simulink model "CM690A_HwAg0Meas"  (R2013b)
settings: Solver=FixedStepDiscrete  SolverMode=SingleTasking  StartTime=0.0  StopTime=22  FixedStep=0.002  RelTol=1e-3
undefined symbols (not defined in the file): ELECGLBPRM_DEGPERREV_DEGPERREV_F32, ELECGLBPRM_HWAGCENTROFFS_HWDEG_F32, ELECGLBPRM_HWAGSATNLOWRLIM_HWDEG_F32, ELECGLBPRM_HWAGSATNUPPRLIM_HWDEG_F32, ELECGLBPRM_HWAGSCA_ULS_F32, ELECGLBPRM_HWAGSPURGEARRAT_ULS_F32, ELECGLBPRM_HWAGSPURTORINGGEARRATSNSR0_ULS_F32, ELECGLBPRM_HWAGSPURTORINGGEARRATSNSR1_ULS_F32, ELECGLBPRM_NOFLT_CNT_U08, ELECGLBPRM_OFFSTRIMNOTPRFMD_CNT_U08, ELECGLBPRM_PRTCLFLT_CNT_U08, ELECGLBPRM_SKIPSTEPFLT_CNT_U08, ELECGLBPRM_SNSRINTFLT_CNT_U08, ELECGLBPRM_VRNRERRFLT_CNT_U08, FLTINJ_HWAG0MEAS_HWAG0, FLTINJ_HWAG0MEAS_TESTOK, HwAg0IfFlt, HwAg0MeasHwAg0IfFltFailStep, HwAg0MeasHwAg0IfFltPassStep, HwAg0MeasHwAg0Snsr0PrtclFltFailStep, HwAg0MeasHwAg0Snsr0PrtclFltPassStep, HwAg0MeasHwAg0Snsr1PrtclFltFailStep, HwAg0MeasHwAg0Snsr1PrtclFltPassStep, HwAg0MeasSnsr0Rev, HwAg0MeasSnsr1Rev, HwAg0MeasStep, HwAg0MeasVrnrErrThd, HwAg0MfgFlt, HwAg0Snsr0PrtclFlt, HwAg0Snsr1PrtclFlt, HWAG10THTOOTHTRIG_CNT_U08, HWAG11THTOOTHTRIG_CNT_U08, NtcSts1, sigbuilder_block, SigQlfr1
libraries: simulink x30, NxtrNvM x3
(part 1 of 5)
settings Model: Creator=CZ68DS  LastModifiedBy=CZ68DS
settings SolverCC: PositivePriorityOrder=on  AutoInsertRateTranBlk=on  InsertRTBMode=Always
settings DataIOCC: LimitDataPoints=off  SaveFormat=Structure  ReturnWorkspaceOutputs=on
settings OptimizationCC: BlockReduction=off  InlineParams=on  ZeroExternalMemoryAtStartup=off  ZeroInternalMemoryAtStartup=off  OptimizeModelRefInitCode=on  LifeSpan=1
settings DebuggingCC: SignalInfNanChecking=error  SignalRangeChecking=warning  ReadBeforeWriteMsg=EnableAllAsWarning  WriteAfterWriteMsg=EnableAllAsWarning  WriteAfterReadMsg=EnableAllAsWarning  UnderspecifiedInitializationDetection=Simplified  MergeDetectMultiDrivingBlocksExec=error  SolverPrmCheckMsg=error  InheritedTsInSrcMsg=error  MultiTaskDSMMsg=warning  SingleTaskRateTransMsg=error  TasksWithSamePriorityMsg=error  SigSpecEnsureSampleTimeMsg=error  CheckMatrixSingularityMsg=error  ParameterUnderflowMsg=error  ParameterPrecisionLossMsg=error  ParameterTunabilityLossMsg=error  FixptConstUnderflowMsg=warning  FixptConstOverflowMsg=warning  FixptConstPrecisionLossMsg=warning  VectorMatrixConversionMsg=error  SignalLabelMismatchMsg=error  UnconnectedInputMsg=error  UnconnectedOutputMsg=error  UnconnectedLineMsg=error  SFcnCompatibilityMsg=error  FrameProcessingCompatibilityMsg=error  UniqueDataStoreMsg=warning  BusObjectLabelMismatch=error  RootOutportRequireBusObject=error  AssertControl=DisableAll  ModelReferenceIOMsg=error  ModelReferenceVersionMismatchMessage=warning  ModelReferenceIOMismatchMessage=error  ModelReferenceDataLoggingMessage=error  StateNameClashWarn=warning  StrictBusMsg=ErrorOnBusTreatedAsVector  NonBusSignalsTreatedAsBus=error  SFUnexpectedBacktrackingDiag=error  SFInvalidInputDataAccessInChartInitDiag=error  SFNoUnconditionalDefaultTransitionDiag=error  SFTransitionOutsideNaturalParentDiag=error  SFUnconditionalTransitionShadowingDiag=error  SFUndirectedBroadcastEventsDiag=error
settings HardwareCC: ProdEndianess=LittleEndian  ProdHWDeviceType=Texas Instruments->TMS470
settings ModelReferenceCC: ModelReferenceNumInstancesAllowed=Single
settings RTWCC: SystemTargetFile=autosar.tlc  GenCodeOnly=on  TemplateMakefile=ert_default_tmf  Description=AUTOSAR  GenerateReport=on  ProcessScript=autosar_make_rtw_hook  LaunchReport=on
settings CodeAppCC: GenerateComments=off  IgnoreCustomStorageClasses=off  CustomSymbolStrType=$N$R$M  CustomSymbolStrBlkIO=$N$M  SimulinkBlockComments=off
settings STFCustomTargetCC: CodeReplacementLibrary=C89/C90 (ANSI)  ParMdlRefBuildCompliant=on  CompOptLevelCompliant=on  IncludeMdlTerminateFcn=off  CombineOutputUpdateFcns=on  SuppressErrorStatus=on  ERTFirstTimeCompliant=on  ERTCustomFileBanners=on  SupportNonFinite=off  SupportComplex=off  SupportContinuousTime=off  SupportNonInlinedSFcns=off  MATLABClassNameForMDSCustomization=Simulink.SoftwareTarget.ERTCustomization  AutosarCompliant=on  GRTInterface=off  SystemTargetFile=autosar.tlc
settings ERTTargetCC: CodeReplacementLibrary=C89/C90 (ANSI)  ConcurrentExecutionCompliant=off  IncludeMdlTerminateFcn=off  SuppressErrorStatus=on  SupportNonFinite=off  SupportComplex=off  ModelStepFunctionPrototypeControlCompliant=off  CPPClassGenCompliant=off  AutosarCompliant=on  InlinedParameterPlacement=NonHierarchical  ERTCustomFileTemplate=example_file_process.tlc  EnableUserReplacementTypes=on

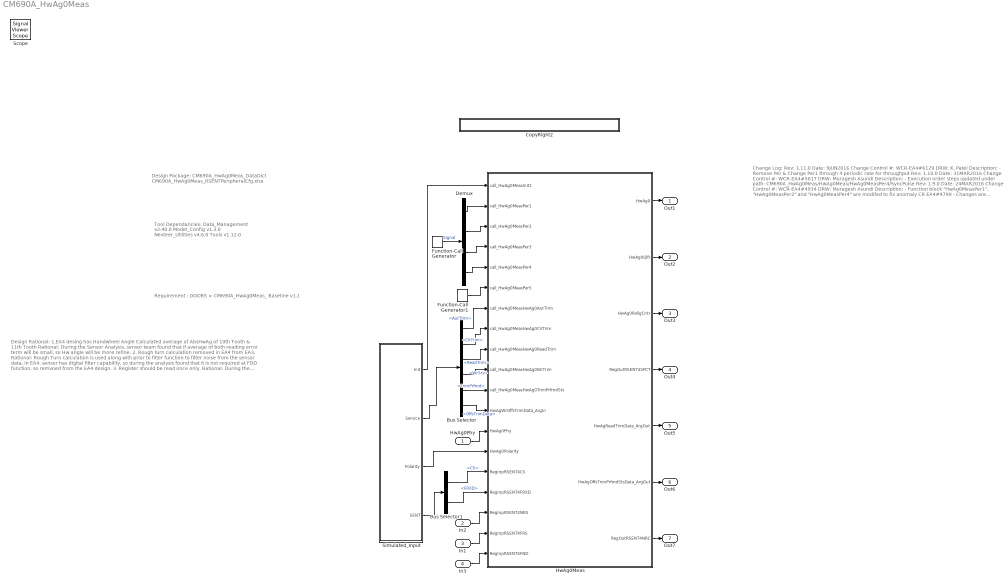
== system CM690A_HwAg0Meas ==
  note: Tool Dependancies:
      |
      | Data_Management v2.40.0
      | Model_Config v1.3.0
      | Nexteer_Utilities v4.6.0
      | Tools v1.12.0
  note: Design Package:
      |
      | CM690A_HwAg0Meas_DataDict
      | CM690A_HwAg0Meas_RSENTPeripheralCfg.xlsx
  note: Requirement :
      |
      | DOORS > CM690A_HwAg0Meas_ Baseline v1.1
  note: Change Log:
      |
      | Rev: 1.11.0
      | Date: 9JUN2016
      | Change Control #: WCR-EA4#6129
      | DRW: K. Patel
      | Description:
      | - Remove Per & Change Per1 through 4 periodic rate for throughput
      |
      | Rev: 1.10.0
      | Date: 31MAR2016
      | Change Control #: WCR-EA4#5017
      | DRW: Muragesh Asundi
      | Description:
      | - Execution order steps updated under path:
      |   CM690A_HwAg0Meas/HwAg0Meas/HwAg0MeasPer4/SyncPulse
      |
      | Rev: 1.9.0
      | Date: 24MAR2016
      | Change Control #: WCR-EA4#4934
      | DRW: Muragesh Asundi
      | Description:
      | - Function block "HwAg0MeasPer1", "HwAg0MeasPer2" and "HwAg0MeasPer4" are modifed
      |   to fix anomaly CR EA4#4799
      | - Changes are highlighted in red color
      |
      | Rev: 1.8.0
      | Date: 26FEB2016
      | Change Control #: WCR-EA4#4011
      | DRW: K. Patel
      | Description:
      | - Refer Red Color High lighted Changes.
      |
      | Rev: 1.7.0
      | Date: 19JAN2016
      | Change Control #: WCR-EA4#3380
      | DRW: K. Patel
      | Description:
      | - Refer Red Color High lighted Changes.
      | - "CM690A_HwAg0Meas_RSENTPeripheralCfg.xlsx" change
      | - m file change
      |
      | Rev: 1.6.0
      | Date: 17DEC2015
      | Change Control #: WCR-EA4#2687
      | DRW: K. Patel
      | Description:
      | - Refer Red Color High lighted Changes.
      |
      | Rev: 1.5.0
      | Date: 06OCT2015
      | Change Control #: WCR-EA4#1871, Anomaly:EA4#1856
      | DRW: K. Patel
      | Description:
      | - Skip step Interface fault
      |
      | Rev: 1.4.0
      | Date: 8SEPT2015
      | Change Control #: WCR-EA4#1528, Anomaly:EA4#1354, Anomaly:EA4#1508
      | DRW: K. Patel
      | Description:
      | - Reading Nibble Fix (peripheral register configuration change)
      | - Cleaning CS register before SPCT
      | - Sensor Synchronization logic added
      |
      | Rev: 1.3.0
      | Date: 11AUG2015
      | Change Control #: WCR-EA4#1240, Anomaly:EA4#1206
      | DRW: K. Patel
      | Description:
      | - Correction m file
      | - Model Correction
      |
      | Rev: 1.2.0
      | Date: 07JUL2015
      | Change Control #: WCR-EA4#1038
      | DRW: K. Patel
      | Description:
      | - Add RollOver Mode Function, skip step rollover
      | - Polarity Unit Corrected in m file
      |
      | Rev: 1.1.0
      | Date: 26JUN2015
      | Change Control #: WCR-EA4#978
      | DRW: K. Patel
      | Description:
      | - Removed Fault injection from Per4, copy paste error from Per3
      | - Constant define as global
      | - Init function Timer implemented
      |
      | Rev: 1.0.0
      | Date: 23JUN2015
      | Change Control #: WCR-EA4#682
      | DRW: K. Patel
      | Description:
      | - Initial Release
      |
      | DRW: Keyur Patel
      | Scope:
      | - Model intent to implement EA4 SENT4 based Digital HandWheel Angle implementation for T1xx.
      |    model runs at different function rate:
      |       1) Init - Configure Peripheral
      |       2) 4ms - Per1 & Per2 use for SENT Trigger
      |       3) 4ms - Per3 Read SENT Data from 10 Tooth & Protocol Fault
      |       4) 4ms - Per4 Read SENT Data from 11 Tooth & Protocol Fault
      |       5) 4ms - Per5 Final HwAg calculation
      |       6) 100ms - Per6 Trim Not Performed evaluation
      |       7) Event Trim Service - Auto, Clear, Write, Read, Trim Performed Status
      | - Fault Injection added
      | - Copyright Blocks added to each layer
  note: Design Rational:
      |
      | 1.EA4 desing has Handwheel Angle Calculated average of AbsHwAg of 10th Tooth &  11th Tooth
      | Rational: During the Sensor Analysis, sensor team found that if average of both reading error term
      | will be small, so Hw angle will be more refine.
      |
      | 2. Rough turn calculation removed in EA4 from EA3.
      | Rational: Rough Turn calculation is used along with prior to filter function to filter noise from the
      | sensor data, in EA4, sensor has digital filter capability, so
      | during the analysis found that it is not required at FDD function, so remvoed from the EA4 design.
      |
      | 3. Register should be read once only.
      | Rational: During the troubleshooting found that when you read message, it will wipe data too.
      | In order to protect the data getting wiped out, it should be read only one time.
      |
      | 4. HwAg0MeasInit2 should be scheduled before Port Config and Port Pin default set to high
      | Rational:
      | Problem: After Multiple approximately 10 power cycle, One of the Handwheel Angle
      | (HwAg0 or HwAg1) seems freeze. Random Issue behaviour.
      |
      | Observation :
      | - 10th tooth and 11th tooth, both dies are sending SENT messages at same time,
      | when first trigger happen and next trigger no one respond.
      |
      | - HwAg sensor runs self test diagnostic at the start up. It might take 40ms to 50ms.
      | - As power applied, SENT bidirectional IO line, stays high until port configuration happen,
      | which takes about 40ms to 50ms. After this stage, it will pull the line low until RTE SENT
      |  Init function happen.  SENT Init will pull line high again.
      |
      | Potential Solution: Test Performed 25 Ignition cycle and verified.
      | Bidirectional IO line, kept high till periodic or make sure they stay high for at least
      | 100ms, seems HwAg didn't freeze & Sensor Trigger Mechanism need to fix
      |
      | 5. RSENTxNRS checked before write RSENTxSPCT
      | Rational: RSENTxNRS gets clear, when RSENTxNRC bit field register is set
      | RSENTxNRC is bit field of RSENTxCSC. During the analysis found that
      | even though we write RSENTxCSC all bit and wait for RSENTxCS, Bit Field
      | RSENTxNRS didn't clear. If RSENTxNRS is set then writing RSENTxSPCT,
      | Peripheral will not output Pulse.
      |
      | Also found that RSENTxCS didn't clear itself, so need to always clear after
      | read message.
      |
      | 6. RSENTxSPCT need to write first to verify RSENTxNRS status
      | Rational : As per the Renesas User's hardware manual v1.0 -
      | Section 19 -SPC function, "Writing to RSENTnSPCT.TLL requests a
      | SPC trigger transmission. After writing to RSENTnSPCT.TLL, the CPU
      | should read RSENTnCS.NRS to check whether the previous request was
      | completed or not."
      |
      | 7. asm "SYNCM" - Anomaly EA4#3968
      | Rational: During the startup found that if you don't use asm "SYNCM" instruction, RSENT seems
      | doesn't send Per1 trigger, which cause Missing message & incorrect Id sequence error, regardless
      | accessing same peripheral instruction execution back to back
  HwAg0Phy : Inport
  In2 : Inport  Port=2
  In1 : Inport  Port=3
  In3 : Inport  Port=4
  Bus Selector : BusSelector  OutputSignals=AutTrim,ClrTrim,ReadTrim,WrSrv,TrimPrfmd,OffsTrimData
  Bus Selector1 : BusSelector  OutputSignals=CS,FRXD
  CopyRight2 : Subsystem  Description=|  mask(Copyright Information){none=on}
      | Copyright info block.                                               
      |                                                                     
      | Place copyright information at the top of every subsystem in design.
      mask prompts: none "No parameters"
      mask help: Place copyright information at the top of every subsystem in design.
      mask Display:
      | NxtrConf = 'Nexteer Confidential';
      | 
      | sys = bdroot; %handle for the current model ("system")
      | first = get_param(sys,'Created');
      | first = first(end-3:end);  %year is last four digits
      | 
      | last = get_param(sys,'LastModifiedDate');
      | if isempty(last)
      |     last = datestr(now,'yyyy');
      | else
      |     last = last(end-3:end);
      | end
      | 
      | if strcmp(first,last)
      |     fprintf('%s -- Copyright %s Nexteer',NxtrConf,first)
      | else
      |     fprintf('%s -- %s%s- %s Nexteer',NxtrConf,char(169),first,last)
      | end
  Demux : Demux
  Function-Call Generator : simulink/Ports & Subsystems/Function-Call Generator  sample_time=0.002  numberOfIterations=1
      settings: AttributesFormatString=%<sample_time>
  Function-Call Generator1 : simulink/Ports & Subsystems/Function-Call Generator  sample_time=0.100  numberOfIterations=1
  HwAg0Meas : Subsystem  RequirementInfo={} %GIDa_1b511019_32d3_4208_ad3f_5416ab2f5672
  Simulated_Input : Subsystem  Description=Do not Code this block
      settings: AttributesFormatString=%<Description>
  Out1 : Outport
  Out2 : Outport  Port=2
  Out3 : Outport  Port=3
  Out4 : Outport  Port=4
  Out5 : Outport  Port=5
  Out6 : Outport  Port=6
  Out7 : Outport  Port=7
  Scope : SignalViewerScope  IOType=viewer  SampleTime=-1  RefreshTime=0.035000
      settings: YMin=-10  YMax=10
  wires:
  Function-Call Generator/1 -> Demux/1  "Signal"
  HwAg0Meas/1(HwAg0) -> Out1/1
  Demux/1 -> HwAg0Meas/2(call_HwAg0MeasPer1)
  Demux/2 -> HwAg0Meas/3(call_HwAg0MeasPer2)
  Demux/3 -> HwAg0Meas/4(call_HwAg0MeasPer3)
  Demux/4 -> HwAg0Meas/5(call_HwAg0MeasPer4)
  Function-Call Generator1/1 -> HwAg0Meas/6(call_HwAg0MeasPer5)
  Simulated_Input/3(Polarity) -> HwAg0Meas/14(HwAg0Polarity)
  HwAg0Meas/2(HwAg0Qlfr) -> Out2/1
  HwAg0Meas/3(HwAg0RollgCntr) -> Out3/1
  HwAg0Meas/4(RegOutRSENT4SPCT) -> Out4/1
  HwAg0Meas/5(HwAgReadTrimData_ArgOut) -> Out5/1
  HwAg0Meas/6(HwAgOffsTrimPrfmdStsData_ArgOut) -> Out6/1
  Simulated_Input/2(Service) -> Bus Selector/1
  Bus Selector/1 -> HwAg0Meas/7(call_HwAg0MeasHwAg0AutTrim)  "<AutTrim>"
  Bus Selector/2 -> HwAg0Meas/8(call_HwAg0MeasHwAg0ClrTrim)  "<ClrTrim>"
  Bus Selector/3 -> HwAg0Meas/9(call_HwAg0MeasHwAg0ReadTrim)  "<ReadTrim>"
  Bus Selector/4 -> HwAg0Meas/10(call_HwAg0MeasHwAg0WrTrim)  "<WrSrv>"
  Bus Selector/5 -> HwAg0Meas/11(call_HwAg0MeasHwAg0TrimPrfmdSts)  "<TrimPrfmd>"
  Bus Selector/6 -> HwAg0Meas/12(HwAgWrOffsTrimData_ArgIn)  "<OffsTrimData>"
  Simulated_Input/1(Init) -> HwAg0Meas/1(call_HwAg0MeasInit1)
  Simulated_Input/4(SENT) -> Bus Selector1/1
  HwAg0Phy/1 -> HwAg0Meas/13(HwAg0Phy)
  Bus Selector1/1 -> HwAg0Meas/15(RegInpRSENT4CS)  "<CS>"
  Bus Selector1/2 -> HwAg0Meas/16(RegInpRSENT4FRXD)  "<FRXD>"
  In2/1 -> HwAg0Meas/17(RegInpRSENT4NRS)
  HwAg0Meas/7(RegOutRSENT4NRC) -> Out7/1
  In3/1 -> HwAg0Meas/19(RegInpRSENT4FND)
  In1/1 -> HwAg0Meas/18(RegInpRSENT4FRS)

== system CM690A_HwAg0Meas/CopyRight2 ==

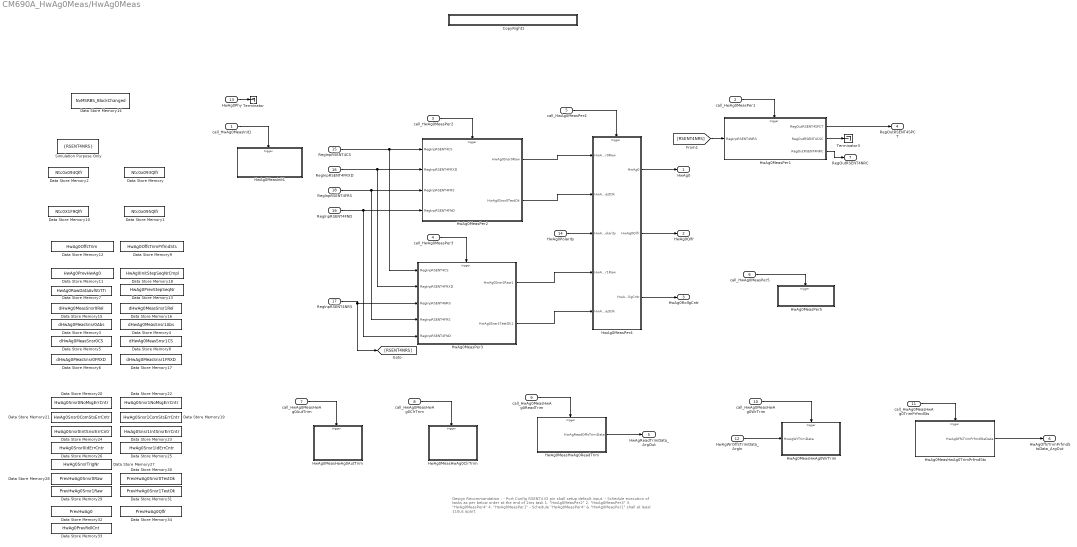
== system CM690A_HwAg0Meas/HwAg0Meas ==
  note: Design Recommandation :
      |
      | - Port Config RSENT4 IO pin shall setup default input.
      | - Schedule execution of tasks as per below order at the end of 2ms task
      |
      |    1.  "HwAg0MeasPer2"
      |    2.  "HwAg0MeasPer3"
      |    3.  "HwAg0MeasPer4"
      |    4.  "HwAg0MeasPer1"
      |
      | - Schedule  "HwAg0MeasPer4" & "HwAg0MeasPer1"  shall at least 110us apart.
  call_HwAg0MeasInit1 : Inport
  call_HwAg0MeasPer1 : Inport  Description=2ms  Port=2
      settings: AttributesFormatString=%<Description>
  call_HwAg0MeasPer2 : Inport  Description=2ms  Port=3
      settings: AttributesFormatString=%<Description>
  call_HwAg0MeasPer3 : Inport  Description=2ms  Port=4
      settings: AttributesFormatString=%<Description>
  call_HwAg0MeasPer4 : Inport  Description=2ms  Port=5
      settings: AttributesFormatString=%<Description>
  call_HwAg0MeasPer5 : Inport  Description=100ms  Port=6
      settings: AttributesFormatString=%<Description>
  call_HwAg0MeasHwAg0AutTrim : Inport  Description=Event  Port=7
      settings: AttributesFormatString=%<Description>
  call_HwAg0MeasHwAg0ClrTrim : Inport  Description=Event  Port=8
      settings: AttributesFormatString=%<Description>
  call_HwAg0MeasHwAg0ReadTrim : Inport  Description=Event  Port=9
      settings: AttributesFormatString=%<Description>
  call_HwAg0MeasHwAg0WrTrim : Inport  Description=Event  Port=10
      settings: AttributesFormatString=%<Description>
  call_HwAg0MeasHwAg0TrimPrfmdSts : Inport  Description=Event  Port=11
      settings: AttributesFormatString=%<Description>
  HwAgWrOffsTrimData_ArgIn : Inport  Port=12
  HwAg0Phy : Inport  Port=13
  HwAg0Polarity : Inport  Port=14  OutDataTypeStr=int8
  RegInpRSENT4CS : Inport  Port=15
  RegInpRSENT4FRXD : Inport  Port=16
  RegInpRSENT4NRS : Inport  Port=17
  RegInpRSENT4FRS : Inport  Port=18
  RegInpRSENT4FND : Inport  Port=19
  CopyRight1 : Subsystem  Description=|  mask(Copyright Information){none=on}
      | Copyright info block.                                               
      |                                                                     
      | Place copyright information at the top of every subsystem in design.
      mask prompts: none "No parameters"
      mask help: Place copyright information at the top of every subsystem in design.
      mask Display:
      | NxtrConf = 'Nexteer Confidential';
      | 
      | sys = bdroot; %handle for the current model ("system")
      | first = get_param(sys,'Created');
      | first = first(end-3:end);  %year is last four digits
      | 
      | last = get_param(sys,'LastModifiedDate');
      | if isempty(last)
      |     last = datestr(now,'yyyy');
      | else
      |     last = last(end-3:end);
      | end
      | 
      | if strcmp(first,last)
      |     fprintf('%s -- Copyright %s Nexteer',NxtrConf,first)
      | else
      |     fprintf('%s -- %s%s- %s Nexteer',NxtrConf,char(169),first,last)
      | end
  Data Store Memory11 : DataStoreMemory  DataStoreName=HwAg0PrevHwAg0  ReadBeforeWriteMsg=warning  WriteAfterWriteMsg=warning  WriteAfterReadMsg=warning  StateMustResolveToSignalObject=on
  Data Store Memory12 : DataStoreMemory  DataStoreName=HwAg0OffsTrim  ReadBeforeWriteMsg=warning  WriteAfterWriteMsg=warning  WriteAfterReadMsg=warning
  Data Store Memory13 : DataStoreMemory  DataStoreName=HwAg0PrevStepSeqNr  ReadBeforeWriteMsg=warning  WriteAfterWriteMsg=warning  WriteAfterReadMsg=warning  StateMustResolveToSignalObject=on
  Data Store Memory14 : DataStoreMemory  Description=|  DataStoreName=NvMSRBS_BlockChanged  ReadBeforeWriteMsg=warning  WriteAfterWriteMsg=warning  WriteAfterReadMsg=warning
      | Simulation Purpose Only.
      | Do Not Code this block
      | NVM Manager Owns this requirement
      settings: AttributesFormatString=%<Description>
  Data Store Memory15 : DataStoreMemory  DataStoreName=dHwAg0MeasSnsr0Rel  ReadBeforeWriteMsg=warning  WriteAfterWriteMsg=warning  WriteAfterReadMsg=warning  StateMustResolveToSignalObject=on
  Data Store Memory16 : DataStoreMemory  DataStoreName=dHwAg0MeasSnsr1Rel  ReadBeforeWriteMsg=warning  WriteAfterWriteMsg=warning  WriteAfterReadMsg=warning  StateMustResolveToSignalObject=on
  Data Store Memory17 : DataStoreMemory  DataStoreName=dHwAg0MeasSnsr1FRXD  ReadBeforeWriteMsg=warning  WriteAfterWriteMsg=warning  WriteAfterReadMsg=warning  StateMustResolveToSignalObject=on
  Data Store Memory18 : DataStoreMemory  DataStoreName=HwAg0InitStepSeqNrCmpl  ReadBeforeWriteMsg=warning  WriteAfterWriteMsg=warning  WriteAfterReadMsg=warning  StateMustResolveToSignalObject=on
  Data Store Memory19 : DataStoreMemory  DataStoreName=HwAg0Snsr1ComStsErrCntr  ReadBeforeWriteMsg=warning  WriteAfterWriteMsg=warning  WriteAfterReadMsg=warning  StateMustResolveToSignalObject=on
  Data Store Memory20 : DataStoreMemory  DataStoreName=HwAg0Snsr0NoMsgErrCntr  ReadBeforeWriteMsg=warning  WriteAfterWriteMsg=warning  WriteAfterReadMsg=warning  StateMustResolveToSignalObject=on
  Data Store Memory21 : DataStoreMemory  DataStoreName=HwAg0Snsr0ComStsErrCntr  ReadBeforeWriteMsg=warning  WriteAfterWriteMsg=warning  WriteAfterReadMsg=warning  StateMustResolveToSignalObject=on
  Data Store Memory22 : DataStoreMemory  DataStoreName=HwAg0Snsr1NoMsgErrCntr  ReadBeforeWriteMsg=warning  WriteAfterWriteMsg=warning  WriteAfterReadMsg=warning  StateMustResolveToSignalObject=on
  Data Store Memory23 : DataStoreMemory  DataStoreName=HwAg0Snsr1IntSnsrErrCntr  ReadBeforeWriteMsg=warning  WriteAfterWriteMsg=warning  WriteAfterReadMsg=warning  StateMustResolveToSignalObject=on
  Data Store Memory24 : DataStoreMemory  DataStoreName=HwAg0Snsr0IntSnsrErrCntr  ReadBeforeWriteMsg=warning  WriteAfterWriteMsg=warning  WriteAfterReadMsg=warning  StateMustResolveToSignalObject=on
  Data Store Memory25 : DataStoreMemory  DataStoreName=HwAg0Snsr1IdErrCntr  ReadBeforeWriteMsg=warning  WriteAfterWriteMsg=warning  WriteAfterReadMsg=warning  StateMustResolveToSignalObject=on
  Data Store Memory26 : DataStoreMemory  DataStoreName=HwAg0Snsr0IdErrCntr  ReadBeforeWriteMsg=warning  WriteAfterWriteMsg=warning  WriteAfterReadMsg=warning  StateMustResolveToSignalObject=on
  Data Store Memory27 : DataStoreMemory  DataStoreName=HwAg0SnsrTrigNr  ReadBeforeWriteMsg=warning  WriteAfterWriteMsg=warning  WriteAfterReadMsg=warning  StateMustResolveToSignalObject=on
  Data Store Memory28 : DataStoreMemory  DataStoreName=PrevHwAg0Snsr0Raw  ReadBeforeWriteMsg=warning  WriteAfterWriteMsg=warning  WriteAfterReadMsg=warning  StateMustResolveToSignalObject=on
  Data Store Memory29 : DataStoreMemory  DataStoreName=PrevHwAg0Snsr1Raw  ReadBeforeWriteMsg=warning  WriteAfterWriteMsg=warning  WriteAfterReadMsg=warning  StateMustResolveToSignalObject=on
  Data Store Memory3 : DataStoreMemory  DataStoreName=dHwAg0MeasSnsr0Abs  ReadBeforeWriteMsg=warning  WriteAfterWriteMsg=warning  WriteAfterReadMsg=warning  StateMustResolveToSignalObject=on
  Data Store Memory30 : DataStoreMemory  DataStoreName=PrevHwAg0Snsr0TestOk  ReadBeforeWriteMsg=warning  WriteAfterWriteMsg=warning  WriteAfterReadMsg=warning  StateMustResolveToSignalObject=on
  Data Store Memory31 : DataStoreMemory  DataStoreName=PrevHwAg0Snsr1TestOk  ReadBeforeWriteMsg=warning  WriteAfterWriteMsg=warning  WriteAfterReadMsg=warning  StateMustResolveToSignalObject=on
  Data Store Memory32 : DataStoreMemory  DataStoreName=PrevHwAg0  ReadBeforeWriteMsg=warning  WriteAfterWriteMsg=warning  WriteAfterReadMsg=warning  StateMustResolveToSignalObject=on
  Data Store Memory33 : DataStoreMemory  DataStoreName=HwAg0PrevRollCnt  ReadBeforeWriteMsg=warning  WriteAfterWriteMsg=warning  WriteAfterReadMsg=warning  StateMustResolveToSignalObject=on
  Data Store Memory34 : DataStoreMemory  DataStoreName=PrevHwAg0Qlfr  ReadBeforeWriteMsg=warning  WriteAfterWriteMsg=warning  WriteAfterReadMsg=warning  InitialValue=SigQlfr1.SIGQLFR_NORES  OutDataTypeStr=Enum: SigQlfr1  StateMustResolveToSignalObject=on
  Data Store Memory4 : DataStoreMemory  DataStoreName=dHwAg0MeasSnsr1Abs  ReadBeforeWriteMsg=warning  WriteAfterWriteMsg=warning  WriteAfterReadMsg=warning  StateMustResolveToSignalObject=on
  Data Store Memory5 : DataStoreMemory  DataStoreName=dHwAg0MeasSnsr0CS  ReadBeforeWriteMsg=warning  WriteAfterWriteMsg=warning  WriteAfterReadMsg=warning  StateMustResolveToSignalObject=on
  Data Store Memory6 : DataStoreMemory  DataStoreName=dHwAg0MeasSnsr0FRXD  ReadBeforeWriteMsg=warning  WriteAfterWriteMsg=warning  WriteAfterReadMsg=warning  StateMustResolveToSignalObject=on
  Data Store Memory7 : DataStoreMemory  DataStoreName=HwAg0RawDataAvlStrtTi  ReadBeforeWriteMsg=warning  WriteAfterWriteMsg=warning  WriteAfterReadMsg=warning  StateMustResolveToSignalObject=on
  Data Store Memory8 : DataStoreMemory  DataStoreName=dHwAg0MeasSnsr1CS  ReadBeforeWriteMsg=warning  WriteAfterWriteMsg=warning  WriteAfterReadMsg=warning  StateMustResolveToSignalObject=on
  Data Store Memory9 : DataStoreMemory  DataStoreName=HwAg0OffsTrimPrfmdSts  ReadBeforeWriteMsg=warning  WriteAfterWriteMsg=warning  WriteAfterReadMsg=warning
  Data Store Memory : DataStoreMemory  DataStoreName=Ntc0x093Qlfr  ReadBeforeWriteMsg=warning  WriteAfterWriteMsg=warning  WriteAfterReadMsg=warning  OutDataTypeStr=uint8
      settings: AttributesFormatString=|
      | Simulation Purpose Only.
      | Do Not Code this block
      | Diagnostic Manager Owns this requirement
  Data Store Memory1 : DataStoreMemory  DataStoreName=Ntc0x095Qlfr  ReadBeforeWriteMsg=warning  WriteAfterWriteMsg=warning  WriteAfterReadMsg=warning  OutDataTypeStr=uint8
      settings: AttributesFormatString=|
      | Simulation Purpose Only.
      | Do Not Code this block
      | Diagnostic Manager Owns this requirement
  Data Store Memory10 : DataStoreMemory  DataStoreName=Ntc0X1F9Qlfr  ReadBeforeWriteMsg=warning  WriteAfterWriteMsg=warning  WriteAfterReadMsg=warning  OutDataTypeStr=uint8
      settings: AttributesFormatString=|
      | Simulation Purpose Only.
      | Do Not Code this block
      | Diagnostic Manager Owns this requirement
  Data Store Memory2 : DataStoreMemory  DataStoreName=Ntc0x094Qlfr  ReadBeforeWriteMsg=warning  WriteAfterWriteMsg=warning  WriteAfterReadMsg=warning  OutDataTypeStr=uint8
      settings: AttributesFormatString=|
      | Simulation Purpose Only.
      | Do Not Code this block
      | Diagnostic Manager Owns this requirement
  HwAg0MeasHwAg0AutTrim : Subsystem  RequirementInfo={'linktype_rmi_doors' '0000cf45 (/ESG Group/FDD Module Requirements/EA4 Specific/CM690A_HwAg0Meas)' '#CM690A_96' 'true' 'REQ: CM690A_96' '' } %GIDa_ea94ffee_6a60_4ad4_8777_fa2e1209d3e2  TreatAsAtomicUnit=on
  HwAg0MeasHwAg0ClrTrim : Subsystem  RequirementInfo={'linktype_rmi_doors' '0000cf45 (/ESG Group/FDD Module Requirements/EA4 Specific/CM690A_HwAg0Meas)' '#CM690A_94' 'true' 'REQ: CM690A_94' '' } %GIDa_ac4d7135_c09e_4b99_819a_ee37d51d6394  TreatAsAtomicUnit=on
  HwAg0MeasHwAg0ReadTrim : Subsystem  RequirementInfo={'linktype_rmi_doors' '0000cf45 (/ESG Group/FDD Module Requirements/EA4 Specific/CM690A_HwAg0Meas)' '#CM690A_92' 'true' 'REQ: CM690A_92' '' } %GIDa_cdad271c_f4aa_4684_91af_0774478ab1dd  TreatAsAtomicUnit=on
  HwAg0MeasHwAg0TrimPrfmdSts : Subsystem  RequirementInfo={'linktype_rmi_doors' '0000cf45 (/ESG Group/FDD Module Requirements/EA4 Specific/CM690A_HwAg0Meas)' '#CM690A_93' 'true' 'REQ: CM690A_93' '' } %GIDa_f9e60140_9f20_40c9_8f6d_edf000506692  TreatAsAtomicUnit=on
  HwAg0MeasHwAg0WrTrim : Subsystem  RequirementInfo={'linktype_rmi_doors' '0000cf45 (/ESG Group/FDD Module Requirements/EA4 Specific/CM690A_HwAg0Meas)' '#CM690A_95' 'true' 'REQ: CM690A_95' '' } %GIDa_3e323fa6_2ebf_495c_adb5_a3e2347a88cc  TreatAsAtomicUnit=on
  HwAg0MeasInit1 : Subsystem  Priority=1  TreatAsAtomicUnit=on
      settings: AttributesFormatString=Priority=%<Priority>
  HwAg0MeasPer1 : Subsystem  RequirementInfo={'linktype_rmi_doors' '0000cf45 (/ESG Group/FDD Module Requirements/EA4 Specific/CM690A_HwAg0Meas)' '#CM690A_112' 'true' 'REQ: CM690A_112' '' } %GIDa_bc322e89_7505_4ced_bd58_d5630035f58c  TreatAsAtomicUnit=on
  HwAg0MeasPer2 : Subsystem  RequirementInfo={'linktype_rmi_doors' '0000cf45 (/ESG Group/FDD Module Requirements/EA4 Specific/CM690A_HwAg0Meas)' '#CM690A_86' 'true' 'REQ: CM690A_86' '' ; 'linktype_rmi_doors' '0000cf45 (/ESG Group/FDD Module Requirements/EA4 Specific/CM690A_HwAg0Meas)' '#CM690A_39' 'true' 'REQ: CM690A_39' '' } %GIDa_9b2c116c_3a4f_439a_af77_b112da5d765b  TreatAsAtomicUnit=on
  HwAg0MeasPer3 : Subsystem  RequirementInfo={'linktype_rmi_doors' '0000cf45 (/ESG Group/FDD Module Requirements/EA4 Specific/CM690A_HwAg0Meas)' '#CM690A_86' 'true' 'REQ: CM690A_86' '' ; 'linktype_rmi_doors' '0000cf45 (/ESG Group/FDD Module Requirements/EA4 Specific/CM690A_HwAg0Meas)' '#CM690A_55' 'true' 'REQ: CM690A_55' '' } %GIDa_7cda62b4_5588_448d_b03e_99bd27827f7d  TreatAsAtomicUnit=on
  HwAg0MeasPer4 : Subsystem  RequirementInfo={'linktype_rmi_doors' '0000cf45 (/ESG Group/FDD Module Requirements/EA4 Specific/CM690A_HwAg0Meas)' '#CM690A_73' 'true' 'REQ: CM690A_73' '' } %GIDa_d2359c71_dfd5_4281_9f6c_59b61df0ca5b  TreatAsAtomicUnit=on
  HwAg0MeasPer5 : Subsystem  RequirementInfo={'linktype_rmi_doors' '0000cf45 (/ESG Group/FDD Module Requirements/EA4 Specific/CM690A_HwAg0Meas)' '#CM690A_102' 'true' 'REQ: CM690A_102' '' } %GIDa_d0a6efa9_4f14_452b_9991_ec4ccddab763  TreatAsAtomicUnit=on
  Simulation Purpose Only : GotoTagVisibility  GotoTag=RSENT4NRS
  Terminator : Terminator
  Terminator3 : Terminator
  HwAg0 : Outport
  HwAg0Qlfr : Outport  Port=2
  HwAg0RollgCntr : Outport  Port=3
  RegOutRSENT4SPCT : Outport  Port=4
  HwAgReadTrimData_ArgOut : Outport  Port=5
  HwAgOffsTrimPrfmdStsData_ArgOut : Outport  Port=6
  RegOutRSENT4NRC : Outport  Port=7
  wires:
  call_HwAg0MeasPer2/1 -> HwAg0MeasPer2/Trigger
  call_HwAg0MeasInit1/1 -> HwAg0MeasInit1/Trigger
  HwAg0Phy/1 -> Terminator/1
  HwAg0MeasPer4/1(HwAg0) -> HwAg0/1
  HwAg0MeasPer4/2(HwAg0Qlfr) -> HwAg0Qlfr/1
  HwAg0MeasPer4/3(HwAg0RollgCntr) -> HwAg0RollgCntr/1
  call_HwAg0MeasPer3/1 -> HwAg0MeasPer3/Trigger
  call_HwAg0MeasPer4/1 -> HwAg0MeasPer4/Trigger
  HwAg0Polarity/1 -> HwAg0MeasPer4/3(HwAg0Polarity)
  call_HwAg0MeasPer1/1 -> HwAg0MeasPer1/Trigger
  HwAg0MeasPer1/1(RegOutRSENT4SPCT) -> RegOutRSENT4SPCT/1
  call_HwAg0MeasHwAg0AutTrim/1 -> HwAg0MeasHwAg0AutTrim/Trigger
  call_HwAg0MeasHwAg0ClrTrim/1 -> HwAg0MeasHwAg0ClrTrim/Trigger
  call_HwAg0MeasHwAg0ReadTrim/1 -> HwAg0MeasHwAg0ReadTrim/Trigger
  call_HwAg0MeasHwAg0WrTrim/1 -> HwAg0MeasHwAg0WrTrim/Trigger
  call_HwAg0MeasHwAg0TrimPrfmdSts/1 -> HwAg0MeasHwAg0TrimPrfmdSts/Trigger
  HwAgWrOffsTrimData_ArgIn/1 -> HwAg0MeasHwAg0WrTrim/1(HwAgWrTrimData)
  HwAg0MeasHwAg0ReadTrim/1(HwAgReadOffsTrimData) -> HwAgReadTrimData_ArgOut/1
  HwAg0MeasHwAg0TrimPrfmdSts/1(HwAgOffsTrimPrfmdStsData) -> HwAgOffsTrimPrfmdStsData_ArgOut/1
  call_HwAg0MeasPer5/1 -> HwAg0MeasPer5/Trigger
  HwAg0MeasPer2/1(HwAg0Snsr0Raw) -> HwAg0MeasPer4/1(HwAg0Snsr0Raw)
  HwAg0MeasPer2/2(HwAg0Snsr0TestOk) -> HwAg0MeasPer4/2(HwAg0Snsr0TestOk)
  HwAg0MeasPer3/1(HwAg0Snsr1Raw1) -> HwAg0MeasPer4/4(HwAg0Snsr1Raw)
  HwAg0MeasPer3/2(HwAg0Snsr1TestOk1) -> HwAg0MeasPer4/5(HwAg0Snsr1TestOk)
  RegInpRSENT4CS/1 -> HwAg0MeasPer3/1(RegInpRSENT4CS), HwAg0MeasPer2/1(RegInpRSENT4CS)
  RegInpRSENT4FRXD/1 -> HwAg0MeasPer3/2(RegInpRSENT4FRXD), HwAg0MeasPer2/2(RegInpRSENT4FRXD)
  RegInpRSENT4NRS/1 -> HwAg0MeasPer3/3(RegInpRSENT4NRS), [RSENT4NRS]
  RegInpRSENT4FRS/1 -> HwAg0MeasPer3/4(RegInpRSENT4FRS), HwAg0MeasPer2/3(RegInpRSENT4FRS)
  RegInpRSENT4FND/1 -> HwAg0MeasPer3/5(RegInpRSENT4FND), HwAg0MeasPer2/4(RegInpRSENT4FND)
  HwAg0MeasPer1/2(RegOutRSENT4CSC) -> Terminator3/1
  [RSENT4NRS] -> HwAg0MeasPer1/1(RegInpRSENT4NRS)
  HwAg0MeasPer1/3(RegOutRSENT4NRC) -> RegOutRSENT4NRC/1

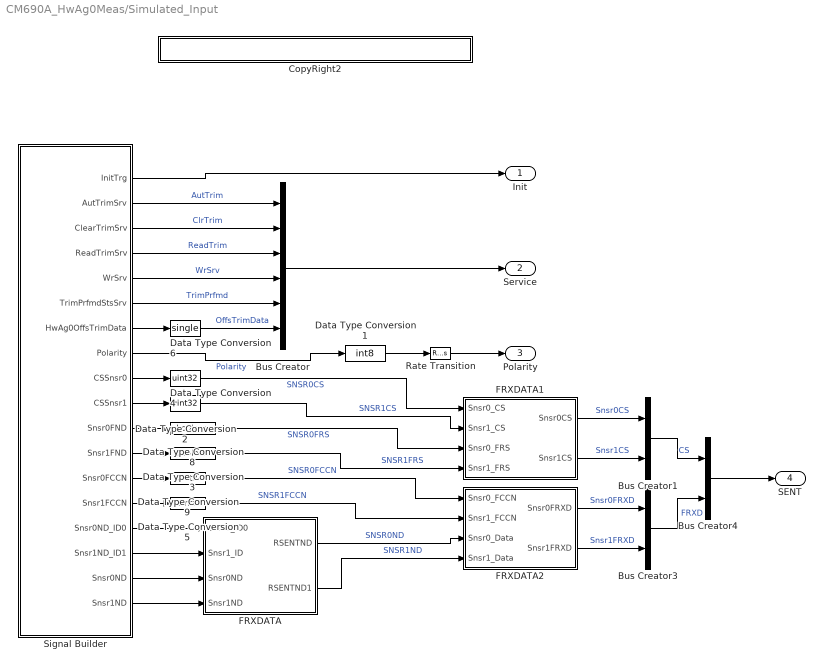
== system CM690A_HwAg0Meas/Simulated_Input ==
  Bus Creator : BusCreator  Inputs=6
  Bus Creator1 : BusCreator  Inputs=2
  Bus Creator3 : BusCreator  Inputs=2
  Bus Creator4 : BusCreator  Inputs=2
  CopyRight2 : Subsystem  Description=|  mask(Copyright Information){none=on}
      | Copyright info block.                                               
      |                                                                     
      | Place copyright information at the top of every subsystem in design.
      mask prompts: none "No parameters"
      mask help: Place copyright information at the top of every subsystem in design.
      mask Display:
      | NxtrConf = 'Nexteer Confidential';
      | 
      | sys = bdroot; %handle for the current model ("system")
      | first = get_param(sys,'Created');
      | first = first(end-3:end);  %year is last four digits
      | 
      | last = get_param(sys,'LastModifiedDate');
      | if isempty(last)
      |     last = datestr(now,'yyyy');
      | else
      |     last = last(end-3:end);
      | end
      | 
      | if strcmp(first,last)
      |     fprintf('%s -- Copyright %s Nexteer',NxtrConf,first)
      | else
      |     fprintf('%s -- %s%s- %s Nexteer',NxtrConf,char(169),first,last)
      | end
  Data Type Conversion1 : DataTypeConversion  OutDataTypeStr=int8
  Data Type Conversion2 : DataTypeConversion  OutDataTypeStr=uint32
  Data Type Conversion3 : DataTypeConversion  OutDataTypeStr=boolean
  Data Type Conversion4 : DataTypeConversion  OutDataTypeStr=uint32
  Data Type Conversion5 : DataTypeConversion  OutDataTypeStr=uint8
  Data Type Conversion6 : DataTypeConversion  OutDataTypeStr=single
  Data Type Conversion8 : DataTypeConversion  OutDataTypeStr=boolean
  Data Type Conversion9 : DataTypeConversion  OutDataTypeStr=uint8
  FRXDATA : Subsystem
  FRXDATA1 : Subsystem
  FRXDATA2 : Subsystem
  Rate Transition : RateTransition
  Signal Builder : Subsystem  Tag=STV Subsys  LoadFcn=sigbuilder_block('load');  StartFcn=sigbuilder_block('start');  StopFcn=sigbuilder_block('stop');  ClipboardFcn=sigbuilder_block('clipboard');  mask(Sigbuilder block){}
      mask help: Simulink:masks:SigbuilderBlock_MD
      mask init:
      | if ~strcmp(get_param(bdroot(gcbh),'SimulationStatus'),'stopped') tuvar = sigbuilder_block('maskInit'); end
      settings: CopyFcn=sigbuilder_block('copy');  DeleteFcn=sigbuilder_block('delete');  ModelCloseFcn=sigbuilder_block('modelClose');  PreSaveFcn=sigbuilder_block('preSave');  PauseFcn=sigbuilder_block('pause');  ContinueFcn=sigbuilder_block('continue');  NameChangeFcn=sigbuilder_block('namechange');  OpenFcn=sigbuilder_block('open',[1440 0 1440 753 ]);  CloseFcn=sigbuilder_block('close');
      mask Display: plot(0, 0, 100, 100,[2, 2, 32, 32, 2], [68, 8, 8, 68, 68],[32, 2], [38, 38], [32, 19, 2],[53, 60, 44], [32, 17, 17, 2],[16, 16, 31, 31]);txt = getActiveGroup(gcbh);text(2, 100, txt,'verticalAlignment', 'top');
  Init : Outport
  Service : Outport  Port=2
  Polarity : Outport  Port=3
  SENT : Outport  Port=4
  wires:
  Signal Builder/8(Polarity) -> Data Type Conversion1/1  "Polarity"
  Signal Builder/1(InitTrg) -> Init/1
  Signal Builder/7(HwAg0OffsTrimData) -> Data Type Conversion6/1
  Signal Builder/6(TrimPrfmdStsSrv) -> Bus Creator/5  "TrimPrfmd"
  Signal Builder/5(WrSrv) -> Bus Creator/4  "WrSrv"
  Signal Builder/4(ReadTrimSrv) -> Bus Creator/3  "ReadTrim"
  Signal Builder/3(ClearTrimSrv) -> Bus Creator/2  "ClrTrim"
  Signal Builder/2(AutTrimSrv) -> Bus Creator/1  "AutTrim"
  Signal Builder/10(CSSnsr1) -> Data Type Conversion2/1
  Signal Builder/15(Snsr0ND_ID0) -> FRXDATA/1(Snsr0_ID0)
  Signal Builder/16(Snsr1ND_ID1) -> FRXDATA/2(Snsr1_ID)
  Signal Builder/17(Snsr0ND) -> FRXDATA/3(Snsr0ND)
  Signal Builder/9(CSSnsr0) -> Data Type Conversion4/1
  Signal Builder/11(Snsr0FND) -> Data Type Conversion8/1
  Signal Builder/12(Snsr1FND) -> Data Type Conversion3/1
  Signal Builder/13(Snsr0FCCN) -> Data Type Conversion9/1
  Signal Builder/14(Snsr1FCCN) -> Data Type Conversion5/1
  Signal Builder/18(Snsr1ND) -> FRXDATA/4(Snsr1ND)
  Bus Creator/1 -> Service/1
  FRXDATA/1(RSENTND) -> FRXDATA2/3(Snsr0_Data)  "SNSR0ND"
  FRXDATA/2(RSENTND1) -> FRXDATA2/4(Snsr1_Data)  "SNSR1ND"
  Data Type Conversion1/1 -> Rate Transition/1
  Rate Transition/1 -> Polarity/1
  Data Type Conversion4/1 -> FRXDATA1/1(Snsr0_CS)  "SNSR0CS"
  Data Type Conversion2/1 -> FRXDATA1/2(Snsr1_CS)  "SNSR1CS"
  Data Type Conversion8/1 -> FRXDATA1/3(Snsr0_FRS)  "SNSR0FRS"
  Data Type Conversion3/1 -> FRXDATA1/4(Snsr1_FRS)  "SNSR1FRS"
  Data Type Conversion9/1 -> FRXDATA2/1(Snsr0_FCCN)  "SNSR0FCCN"
  Data Type Conversion5/1 -> FRXDATA2/2(Snsr1_FCCN)  "SNSR1FCCN"
  Data Type Conversion6/1 -> Bus Creator/6  "OffsTrimData"
  FRXDATA1/2(Snsr1CS) -> Bus Creator1/2  "Snsr1CS"
  FRXDATA1/1(Snsr0CS) -> Bus Creator1/1  "Snsr0CS"
  FRXDATA2/1(Snsr0FRXD) -> Bus Creator3/1  "Snsr0FRXD"
  FRXDATA2/2(Snsr1FRXD) -> Bus Creator3/2  "Snsr1FRXD"
  Bus Creator1/1 -> Bus Creator4/1  "CS"
  Bus Creator3/1 -> Bus Creator4/2  "FRXD"
  Bus Creator4/1 -> SENT/1

== system CM690A_HwAg0Meas/HwAg0Meas/CopyRight1 ==

== system CM690A_HwAg0Meas/HwAg0Meas/HwAg0MeasHwAg0AutTrim ==
  function : TriggerPort
  CopyRight2 : Subsystem  Description=|  mask(Copyright Information){none=on}
      | Copyright info block.                                               
      |                                                                     
      | Place copyright information at the top of every subsystem in design.
      mask prompts: none "No parameters"
      mask help: Place copyright information at the top of every subsystem in design.
      mask Display:
      | NxtrConf = 'Nexteer Confidential';
      | 
      | sys = bdroot; %handle for the current model ("system")
      | first = get_param(sys,'Created');
      | first = first(end-3:end);  %year is last four digits
      | 
      | last = get_param(sys,'LastModifiedDate');
      | if isempty(last)
      |     last = datestr(now,'yyyy');
      | else
      |     last = last(end-3:end);
      | end
      | 
      | if strcmp(first,last)
      |     fprintf('%s -- Copyright %s Nexteer',NxtrConf,first)
      | else
      |     fprintf('%s -- %s%s- %s Nexteer',NxtrConf,char(169),first,last)
      | end
  NVM Shadow RAM : DataStoreWrite  RequirementInfo={} %GIDa_c48bf4d8_e676_4fba_a351_533fe7cd0c6e  DataStoreName=HwAg0OffsTrim
  NVM1 Shadow RAM : DataStoreWrite  RequirementInfo={'linktype_rmi_doors' '0000cf45 (/ESG Group/FDD Module Requirements/EA4 Specific/CM690A_HwAg0Meas)' '#CM690A_50' 'true' 'REQ: CM690A_50' '' } %GIDa_a97d023e_c210_4163_b9cc_4aaf2b68072e  DataStoreName=HwAg0OffsTrimPrfmdSts
  PIM : DataStoreRead  Priority=10  DataStoreName=HwAg0PrevHwAg0
      settings: AttributesFormatString=Priority=%<Priority>
  Set : Constant
  Set Ram Block Status : NxtrNvM/Set Ram Block Status  FuncName=Set Ram Block Status  NvMBlockName=HwAg0Offs  VoidFuncRtn=on  BlockChanged_DSN=NvMSRBS_BlockChanged  Return_DSN=NvMSRBS_Return
      settings: AttributesFormatString=%<FuncName>
  Set3 : Constant
  wires:
  PIM/1 -> NVM Shadow RAM/1
  Set/1 -> NVM1 Shadow RAM/1
  Set3/1 -> Set Ram Block Status/1

== system CM690A_HwAg0Meas/HwAg0Meas/HwAg0MeasHwAg0ClrTrim ==
  function : TriggerPort
  Clear1 : Constant  Value=0  OutDataTypeStr=single
  Clear2 : Constant  Value=0
  CopyRight2 : Subsystem  Description=|  mask(Copyright Information){none=on}
      | Copyright info block.                                               
      |                                                                     
      | Place copyright information at the top of every subsystem in design.
      mask prompts: none "No parameters"
      mask help: Place copyright information at the top of every subsystem in design.
      mask Display:
      | NxtrConf = 'Nexteer Confidential';
      | 
      | sys = bdroot; %handle for the current model ("system")
      | first = get_param(sys,'Created');
      | first = first(end-3:end);  %year is last four digits
      | 
      | last = get_param(sys,'LastModifiedDate');
      | if isempty(last)
      |     last = datestr(now,'yyyy');
      | else
      |     last = last(end-3:end);
      | end
      | 
      | if strcmp(first,last)
      |     fprintf('%s -- Copyright %s Nexteer',NxtrConf,first)
      | else
      |     fprintf('%s -- %s%s- %s Nexteer',NxtrConf,char(169),first,last)
      | end
  NVM Shadow RAM : DataStoreWrite  RequirementInfo={} %GIDa_8ccce71d_7994_42b7_8f38_740ca71fc321  DataStoreName=HwAg0OffsTrim
  NVM1 Shadow RAM : DataStoreWrite  RequirementInfo={'linktype_rmi_doors' '0000cf45 (/ESG Group/FDD Module Requirements/EA4 Specific/CM690A_HwAg0Meas)' '#CM690A_50' 'true' 'REQ: CM690A_50' '' } %GIDa_d7bc93a5_b812_40ff_9390_fa70717297a5  DataStoreName=HwAg0OffsTrimPrfmdSts
  Set Ram Block Status : NxtrNvM/Set Ram Block Status  FuncName=Set Ram Block Status  NvMBlockName=HwAg0Offs  VoidFuncRtn=on  BlockChanged_DSN=NvMSRBS_BlockChanged  Return_DSN=NvMSRBS_Return
      settings: AttributesFormatString=%<FuncName>
  Set3 : Constant
  wires:
  Clear1/1 -> NVM Shadow RAM/1
  Clear2/1 -> NVM1 Shadow RAM/1
  Set3/1 -> Set Ram Block Status/1

== system CM690A_HwAg0Meas/HwAg0Meas/HwAg0MeasHwAg0ReadTrim ==
  function : TriggerPort
  CopyRight2 : Subsystem  Description=|  mask(Copyright Information){none=on}
      | Copyright info block.                                               
      |                                                                     
      | Place copyright information at the top of every subsystem in design.
      mask prompts: none "No parameters"
      mask help: Place copyright information at the top of every subsystem in design.
      mask Display:
      | NxtrConf = 'Nexteer Confidential';
      | 
      | sys = bdroot; %handle for the current model ("system")
      | first = get_param(sys,'Created');
      | first = first(end-3:end);  %year is last four digits
      | 
      | last = get_param(sys,'LastModifiedDate');
      | if isempty(last)
      |     last = datestr(now,'yyyy');
      | else
      |     last = last(end-3:end);
      | end
      | 
      | if strcmp(first,last)
      |     fprintf('%s -- Copyright %s Nexteer',NxtrConf,first)
      | else
      |     fprintf('%s -- %s%s- %s Nexteer',NxtrConf,char(169),first,last)
      | end
  NVM Shadow RAM : DataStoreRead  DataStoreName=HwAg0OffsTrim
  HwAgReadOffsTrimData : Outport
  wires:
  NVM Shadow RAM/1 -> HwAgReadOffsTrimData/1

== system CM690A_HwAg0Meas/HwAg0Meas/HwAg0MeasHwAg0TrimPrfmdSts ==
  function : TriggerPort
  CopyRight2 : Subsystem  Description=|  mask(Copyright Information){none=on}
      | Copyright info block.                                               
      |                                                                     
      | Place copyright information at the top of every subsystem in design.
      mask prompts: none "No parameters"
      mask help: Place copyright information at the top of every subsystem in design.
      mask Display:
      | NxtrConf = 'Nexteer Confidential';
      | 
      | sys = bdroot; %handle for the current model ("system")
      | first = get_param(sys,'Created');
      | first = first(end-3:end);  %year is last four digits
      | 
      | last = get_param(sys,'LastModifiedDate');
      | if isempty(last)
      |     last = datestr(now,'yyyy');
      | else
      |     last = last(end-3:end);
      | end
      | 
      | if strcmp(first,last)
      |     fprintf('%s -- Copyright %s Nexteer',NxtrConf,first)
      | else
      |     fprintf('%s -- %s%s- %s Nexteer',NxtrConf,char(169),first,last)
      | end
  Data Store Read1 : DataStoreRead  DataStoreName=HwAg0OffsTrimPrfmdSts
  HwAgOffsTrimPrfmdStsData : Outport
  wires:
  Data Store Read1/1 -> HwAgOffsTrimPrfmdStsData/1

== system CM690A_HwAg0Meas/HwAg0Meas/HwAg0MeasHwAg0WrTrim ==
  HwAgWrTrimData : Inport
  function : TriggerPort
  CopyRight2 : Subsystem  Description=|  mask(Copyright Information){none=on}
      | Copyright info block.                                               
      |                                                                     
      | Place copyright information at the top of every subsystem in design.
      mask prompts: none "No parameters"
      mask help: Place copyright information at the top of every subsystem in design.
      mask Display:
      | NxtrConf = 'Nexteer Confidential';
      | 
      | sys = bdroot; %handle for the current model ("system")
      | first = get_param(sys,'Created');
      | first = first(end-3:end);  %year is last four digits
      | 
      | last = get_param(sys,'LastModifiedDate');
      | if isempty(last)
      |     last = datestr(now,'yyyy');
      | else
      |     last = last(end-3:end);
      | end
      | 
      | if strcmp(first,last)
      |     fprintf('%s -- Copyright %s Nexteer',NxtrConf,first)
      | else
      |     fprintf('%s -- %s%s- %s Nexteer',NxtrConf,char(169),first,last)
      | end
  NVM Shadow RAM : DataStoreWrite  RequirementInfo={} %GIDa_dfafe5ae_08bd_4bd9_b83d_678516e8f399  DataStoreName=HwAg0OffsTrim
  NVM1 Shadow RAM : DataStoreWrite  RequirementInfo={'linktype_rmi_doors' '0000cf45 (/ESG Group/FDD Module Requirements/EA4 Specific/CM690A_HwAg0Meas)' '#CM690A_50' 'true' 'REQ: CM690A_50' '' } %GIDa_43ae7be7_0f33_49ca_abd0_4c14044b69a7  DataStoreName=HwAg0OffsTrimPrfmdSts
  Set : Constant
  Set Ram Block Status : NxtrNvM/Set Ram Block Status  FuncName=Set Ram Block Status  NvMBlockName=HwAg0Offs  VoidFuncRtn=on  BlockChanged_DSN=NvMSRBS_BlockChanged  Return_DSN=NvMSRBS_Return
      settings: AttributesFormatString=%<FuncName>
  Set3 : Constant
  wires:
  Set/1 -> NVM1 Shadow RAM/1
  HwAgWrTrimData/1 -> NVM Shadow RAM/1
  Set3/1 -> Set Ram Block Status/1

== system CM690A_HwAg0Meas/HwAg0Meas/HwAg0MeasInit1 ==
  note: Follow below steps in same order:
      |
      | 1. Enable Configuration mode, RSENT4MDC.OMC = 1U
      | 2. Verify whether peripheral is in Configuration mode RSENT4MST.OMS ==1U and wait till 2us* , it is in configuration mode
      | 3. Configure the SENT Register as per  "CM690A_HwAg0Meas_RSENTPeripheralCfg.xlsx"
      | 4. Enable Operation active mode, RSENT4MDC.OMC = 5U
      | 5. Verify whether peripheral is in Opertation active mode RSENT4MST.OMS ==5U and wait till 2us*, it is in Opertation active mode
      | 6. Client Call "IoHwAb_SetFctPrphlHwAg0"- Port Configuration shall change to output in alternate mode from default input for RSENT4 SPCO IO pin.
      |
      | Note: * - actual minimum is 150ns as per Scott Winder email from Renesas
  function : TriggerPort  TriggerType=falling
  CopyRight2 : Subsystem  Description=|  mask(Copyright Information){none=on}
      | Copyright info block.                                               
      |                                                                     
      | Place copyright information at the top of every subsystem in design.
      mask prompts: none "No parameters"
      mask help: Place copyright information at the top of every subsystem in design.
      mask Display:
      | NxtrConf = 'Nexteer Confidential';
      | 
      | sys = bdroot; %handle for the current model ("system")
      | first = get_param(sys,'Created');
      | first = first(end-3:end);  %year is last four digits
      | 
      | last = get_param(sys,'LastModifiedDate');
      | if isempty(last)
      |     last = datestr(now,'yyyy');
      | else
      |     last = last(end-3:end);
      | end
      | 
      | if strcmp(first,last)
      |     fprintf('%s -- Copyright %s Nexteer',NxtrConf,first)
      | else
      |     fprintf('%s -- %s%s- %s Nexteer',NxtrConf,char(169),first,last)
      | end
  GetRefTmr1MicroSec32bit : Subsystem
      settings: AttributesFormatString=Client Call : Start Time
  GetTiSpan1MicroSec32bit : Subsystem
  IoHwAb_SetFctPrphlHwAg0 : Subsystem
  Terminator1 : Terminator
  wires:
  GetTiSpan1MicroSec32bit/1(TiSpan) -> Terminator1/1
  GetRefTmr1MicroSec32bit/1(RefTmr) -> GetTiSpan1MicroSec32bit/1(RefTmr)

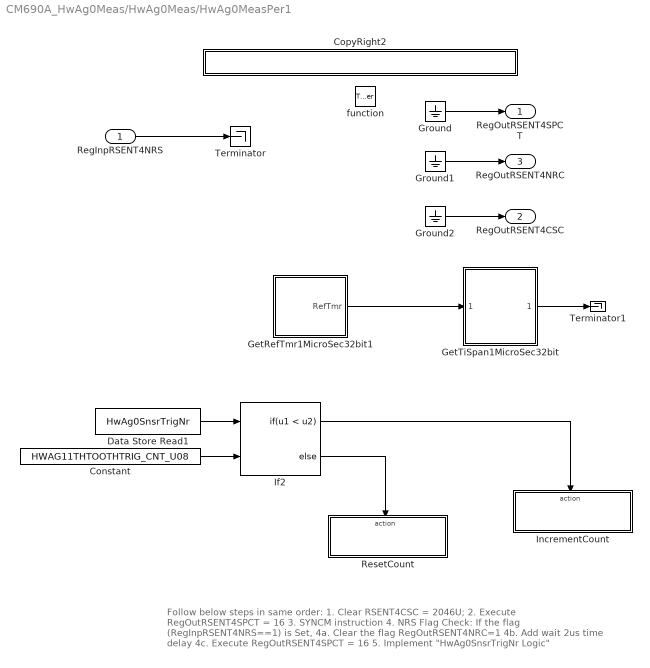
== system CM690A_HwAg0Meas/HwAg0Meas/HwAg0MeasPer1 ==
  note: Follow below steps in same order:
      |
      | 1. Clear RSENT4CSC = 2046U;
      | 2. Execute RegOutRSENT4SPCT = 16
      | 3. SYNCM instruction
      | 4. NRS Flag Check: If the flag (RegInpRSENT4NRS==1) is Set,
      | 	4a. Clear the flag RegOutRSENT4NRC=1
      | 	4b. Add wait 2us time delay
      | 	4c. Execute RegOutRSENT4SPCT = 16
      |
      | 5. Implement "HwAg0SnsrTrigNr Logic"
  RegInpRSENT4NRS : Inport
  function : TriggerPort  TriggerType=function-call
  Constant : Constant  Value=HWAG11THTOOTHTRIG_CNT_U08
      settings: AttributesFormatString=%<Value>.EngVal = 2
  CopyRight2 : Subsystem  Description=|  mask(Copyright Information){none=on}
      | Copyright info block.                                               
      |                                                                     
      | Place copyright information at the top of every subsystem in design.
      mask prompts: none "No parameters"
      mask help: Place copyright information at the top of every subsystem in design.
      mask Display:
      | NxtrConf = 'Nexteer Confidential';
      | 
      | sys = bdroot; %handle for the current model ("system")
      | first = get_param(sys,'Created');
      | first = first(end-3:end);  %year is last four digits
      | 
      | last = get_param(sys,'LastModifiedDate');
      | if isempty(last)
      |     last = datestr(now,'yyyy');
      | else
      |     last = last(end-3:end);
      | end
      | 
      | if strcmp(first,last)
      |     fprintf('%s -- Copyright %s Nexteer',NxtrConf,first)
      | else
      |     fprintf('%s -- %s%s- %s Nexteer',NxtrConf,char(169),first,last)
      | end
  Data Store Read1 : DataStoreRead  DataStoreName=HwAg0SnsrTrigNr
  GetRefTmr1MicroSec32bit1 : Subsystem
      settings: AttributesFormatString=Client Call : Start Time
  GetTiSpan1MicroSec32bit : Subsystem
  Ground : Ground
  Ground1 : Ground
  Ground2 : Ground
  If2 : If  RequirementInfo={} %GIDa_a2f39466_00f8_4ce4_b021_7cb050421b12  NumInputs=2  IfExpression=u1 < u2
  IncrementCount : Subsystem  RequirementInfo={} %GIDa_7fb77453_932a_4b5f_8ef0_60148f555fe8  TreatAsAtomicUnit=on
  ResetCount : Subsystem  RequirementInfo={} %GIDa_5bc77fa9_9f3f_4049_a10d_c3a8d475ec8e  TreatAsAtomicUnit=on
  Terminator : Terminator
  Terminator1 : Terminator
  RegOutRSENT4SPCT : Outport
  RegOutRSENT4CSC : Outport  Port=2
  RegOutRSENT4NRC : Outport  Port=3
  wires:
  Ground/1 -> RegOutRSENT4SPCT/1
  Ground2/1 -> RegOutRSENT4CSC/1
  GetTiSpan1MicroSec32bit/1(TiSpan) -> Terminator1/1
  GetRefTmr1MicroSec32bit1/1(RefTmr) -> GetTiSpan1MicroSec32bit/1(RefTmr)
  Ground1/1 -> RegOutRSENT4NRC/1
  RegInpRSENT4NRS/1 -> Terminator/1
  If2/1 -> IncrementCount/Action
  If2/2 -> ResetCount/Action
  Data Store Read1/1 -> If2/1
  Constant/1 -> If2/2
